simulink model "chapter2_P2"  (R2017a)
settings: Solver=ode1  StartTime=0.0  StopTime=3  FixedStep=0.001  RelTol=1e-3  EnableMultiTasking=on
values from neighbouring files (symbols this model uses):
  K = place(A,B,[pls(1) pls(2) 0 real(pls(1)) ])    [ece486_finalproj1.m]
libraries: c6xlib x2
Description:
  | Real-Time Van der Pol Simulation
  | 
  | This demonstration shows a real-time version of the Simulink(R) Van der Pol
  | simulation demo. This model does not need any external signals, so it does
  | not need any data acquisition hardware or driver. This makes the model ideal
  | for first experiments with Real-Time Windows Target(TM), without need to
  | worry about proper I/O hardware configuration.
  | 
  | How to run this demo:
  | 
  |   1. Build the model using Tools -> Real-Time Workshop -> Build Model.
  |   2. Connect to the real-time code using Simulation -> Connect to target.
  |   3. Start the real-time execution using Simulation -> Start real-time code.
settings Model: SimulationMode=external  ExtModeTrigDuration=50000  Creator=Houska  LastModifiedBy=maherna4
settings DataIOCC: SaveFormat=Array  SignalLoggingSaveFormat=ModelDataLogs  SignalLoggingName=logsOut
settings OptimizationCC: ExpressionDepthLimit=2147483647  InitFltsAndDblsToZero=on  EfficientMapNaN2IntZero=off
settings DebuggingCC: UnderspecifiedInitializationDetection=Classic  MergeDetectMultiDrivingBlocksExec=none  SignalResolutionControl=TryResolveAllWithWarning  FcnCallInpInsideContextMsg=warning  StateNameClashWarn=warning  SFUnexpectedBacktrackingDiag=warning  SFNoUnconditionalDefaultTransitionDiag=warning  SFExecutionAtInitializationDiag=none
settings ModelReferenceCC: PropagateSignalLabelsOutOfModel=off
settings RTWCC: SystemTargetFile=sldrt.tlc  TemplateMakefile=sldrt.tmf  Description=Simulink Desktop Real-Time  RTWCompilerOptimization=on
settings CodeAppCC: MaxIdLength=95
settings SimulinkDesktopRealTimeCC: TargetPreCompLibLocation=C:\MATLABR2017a\toolbox\sldrt\lib\win64  TargetLangStandard=C89/C90 (ANSI)  SupportVariableSizeSignals=off
settings ConfigComp: CovMetricSettings=dw  CovHtmlReporting=on  CovSaveCumulativeToWorkspaceVar=on  CovSaveSingleToWorkspaceVar=on  CovExternalEMLEnable=off  CovSFcnEnable=off

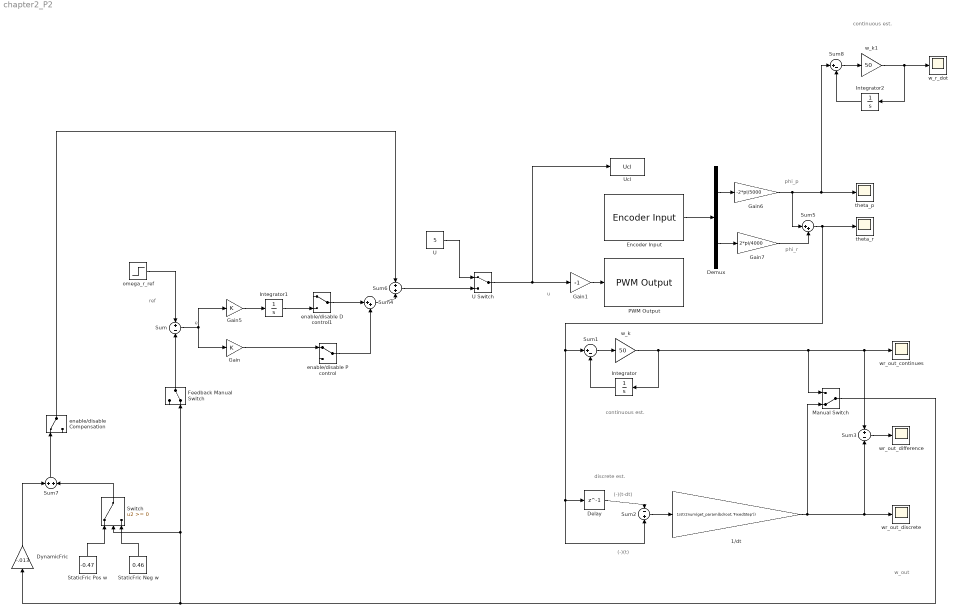
== system chapter2_P2 ==
  note: (-)(t)
  note: w_out
  note: e
  note: u
  note: phi_r
  note: phi_p
  note: discrete est.
  note: continuous est.
  note: (-)(t-dt)
  note: continuous est.
  note: ref
  1/dt : Gain  Gain=1/str2num(get_param(bdroot,'FixedStep'))
  Delay : Delay  DelayLength=1  InitialCondition=0
  Demux : Demux  Outputs=2
  DynamicFric : Gain  Gain=-.013
  Encoder Input : c6xlib/Encoder Input  baseAddr=0x378  channels=[0 1]  sampleTime=str2num(get_param(bdroot, 'FixedStep'))
  Feedback Manual Switch : ManualSwitch  CurrentSetting=0
  Gain : Gain  Gain=K
  Gain1 : Gain  Gain=-1
  Gain5 : Gain  Gain=K
  Gain6 : Gain  Gain=-2*pi/5000
  Gain7 : Gain  Gain=2*pi/4000
  Integrator : Integrator
  Integrator1 : Integrator
  Integrator2 : Integrator
  Manual Switch : ManualSwitch  CurrentSetting=0
  PWM Output : c6xlib/PWM Output  baseAddr=0x378  channels=0  initialOutputs=0  finalOutputs=0  sampleTime=str2num(get_param(bdroot, 'FixedStep'))
  "StaticFric Neg w " : Constant  Value=0.46
  StaticFric Pos w : Constant  Value=-0.47
  Sum : Sum  Inputs=+-
  Sum1 : Sum  Inputs=|+-
  Sum2 : Sum  Inputs=-+
  Sum3 : Sum  Inputs=+-
  Sum4 : Sum  Inputs=|++
  Sum5 : Sum  Inputs=|++
  Sum6 : Sum
  Sum7 : Sum
  Sum8 : Sum  Inputs=|+-
  Switch : Switch
  U : Constant  Value=5
  U Switch : ManualSwitch
  Ucl : ToWorkspace  VariableName=Ucl  SampleTime=-1
  enable/disable Compensation : ManualSwitch
  enable/disable D control1 : ManualSwitch
  enable/disable P control : ManualSwitch
  omega_r_ref : Step  Time=0  After=5  SampleTime=0
  theta_p : Scope
  theta_r : Scope
  w_k : Gain  Gain=50
  w_k1 : Gain  Gain=50
  w_r_dot : Scope
  wr_out_continues : Scope
  wr_out_difference : Scope
  wr_out_discrete : Scope
  wires:
  Demux/1 -> Gain6/1
  enable/disable D control1/1 -> Sum4/1
  w_k/1 -> Manual Switch/1, wr_out_continues/1, Sum3/1, Integrator/1
  Gain/1 -> enable/disable P control/1
  Integrator/1 -> Sum1/2
  Manual Switch/1 -> DynamicFric/1, Switch/2, Feedback Manual Switch/2
  Encoder Input/1 -> Demux/1
  Demux/2 -> Gain7/1
  1/dt/1 -> Manual Switch/2, wr_out_discrete/1, Sum3/2
  enable/disable Compensation/1 -> Sum6/1
  Gain5/1 -> Integrator1/1
  U/1 -> U Switch/1
  Sum2/1 -> 1/dt/1
  Sum6/1 -> U Switch/2
  Sum8/1 -> w_k1/1
  Sum/1 -> Gain5/1, Gain/1
  Gain7/1 -> Sum5/2
  Feedback Manual Switch/1 -> Sum/2
  U Switch/1 -> Gain1/1, Ucl/1
  Switch/1 -> Sum7/2
  Sum3/1 -> wr_out_difference/1
  Delay/1 -> Sum2/1
  Integrator1/1 -> enable/disable D control1/2
  "StaticFric Neg w "/1 -> Switch/3
  Gain6/1 -> Sum8/1, theta_p/1, Sum5/1
  enable/disable P control/1 -> Sum4/2
  DynamicFric/1 -> Sum7/1
  Sum1/1 -> w_k/1
  Sum7/1 -> enable/disable Compensation/1
  Sum5/1 -> theta_r/1, Delay/1, Sum2/2, Sum1/1
  Gain1/1 -> PWM Output/1
  StaticFric Pos w/1 -> Switch/1
  Integrator2/1 -> Sum8/2
  w_k1/1 -> Integrator2/1, w_r_dot/1
  Sum4/1 -> Sum6/2
  omega_r_ref/1 -> Sum/1
